simulink model "nonlinear_model"  (R2018a)
settings: Solver=ode45  StartTime=0.0  StopTime=80  RelTol=1e-3  EnableMultiTasking=on
settings Model: Creator=Lazaros  LastModifiedBy=Li Gen
settings DataIOCC: SaveFormat=Array  Refine=4
settings OptimizationCC: LifeSpan=inf
settings DebuggingCC: UnderspecifiedInitializationDetection=Classic  MergeDetectMultiDrivingBlocksExec=none  SolverPrmCheckMsg=warning  StateNameClashWarn=warning  SFUnexpectedBacktrackingDiag=warning  SFNoUnconditionalDefaultTransitionDiag=warning  SFExecutionAtInitializationDiag=none
settings HardwareCC: ProdBitPerPointer=32  ProdBitPerSizeT=32  ProdBitPerPtrDiffT=32  ProdLargestAtomicFloat=None  ProdIntDivRoundTo=Undefined  ProdEndianess=Unspecified  ProdWordSize=32  ProdHWDeviceType=32-bit Generic
settings ModelReferenceCC: PropagateSignalLabelsOutOfModel=off
settings CodeAppCC: StateflowObjectComments=on
settings GRTTargetCC: TargetLangStandard=C89/C90 (ANSI)  GeneratePreprocessorConditionals=Disable all
settings ConfigComp: CovMetricSettings=dw  CovHtmlReporting=on  CovSaveCumulativeToWorkspaceVar=on  CovSaveSingleToWorkspaceVar=on  CovExternalEMLEnable=off

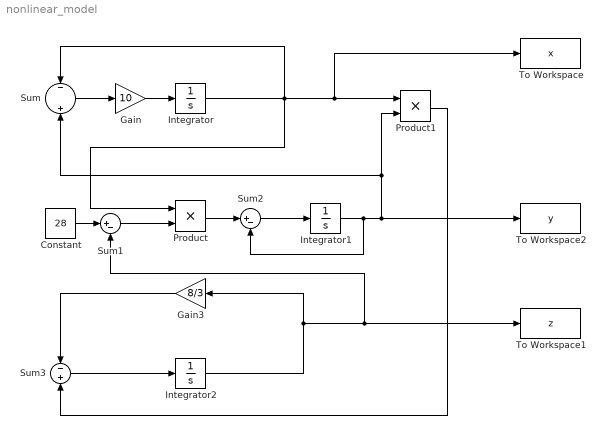
== system nonlinear_model ==
  Constant : Constant  Value=28
  Gain : Gain  Gain=10
  Gain3 : Gain  Gain=8/3
  Integrator : Integrator  InitialCondition=5
  Integrator1 : Integrator  InitialCondition=5
  Integrator2 : Integrator  InitialCondition=5
  Product : Product
  Product1 : Product
  Sum : Sum  Inputs=-|||+
  Sum1 : Sum  Inputs=|+-
  Sum2 : Sum  Inputs=|+-
  Sum3 : Sum  Inputs=-+
  To Workspace : ToWorkspace  VariableName=x  SampleTime=-1
  To Workspace1 : ToWorkspace  VariableName=z  SampleTime=-1
  To Workspace2 : ToWorkspace  VariableName=y  SampleTime=-1
  wires:
  Integrator/1 -> To Workspace/1, Product1/1, Product/1, Sum/1
  Sum/1 -> Gain/1
  Gain/1 -> Integrator/1
  Integrator1/1 -> Sum2/2, To Workspace2/1, Product1/2, Sum/2
  Integrator2/1 -> Gain3/1, To Workspace1/1, Sum1/2
  Sum1/1 -> Product/2
  Product/1 -> Sum2/1
  Sum2/1 -> Integrator1/1
  Sum3/1 -> Integrator2/1
  Gain3/1 -> Sum3/1
  Product1/1 -> Sum3/2
  Constant/1 -> Sum1/1
